simulink model "lugreDenemeFinal"  (R2023b)
settings: Solver=ode23t  StartTime=t_final(1)  StopTime=t_final(end)  FixedStep=1e-3  RelTol=1e-3
values from neighbouring files (symbols this model uses):
  Fc = (v >= 0)*Fc_p + (v < 0)*Fc_n    [frictionModel_20260408.m]    (also in lugreEstTranModel.m = Fc_n; proposed_friction_model.m = params.Fc)
  Fs = (v >= 0)*Fs_p + (v < 0)*Fs_n    [frictionModel_20260408.m]    (also in lugreEstTranModel.m = Fs_n; proposed_friction_model.m = params.Fs)
  vs = vs_n    [lugreEstTranModel.m]    (also in proposed_friction_model.m = params.vs)
undefined symbols (not defined in the file or in its folder): m, sigma_0, sigma_1, sigma_2, v_final
settings Model: Creator=snr  LastModifiedBy=snr

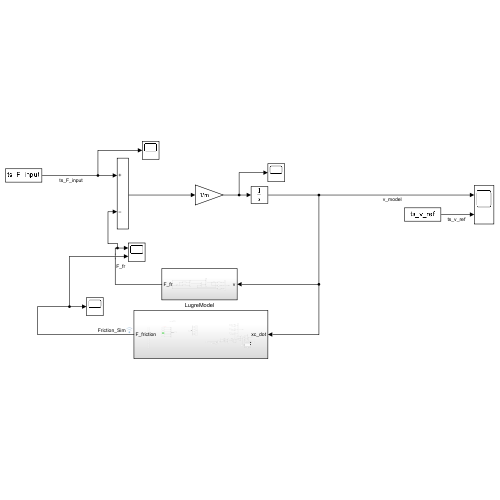
[thumbnail: Simulink's stored preview of the top-level diagram]
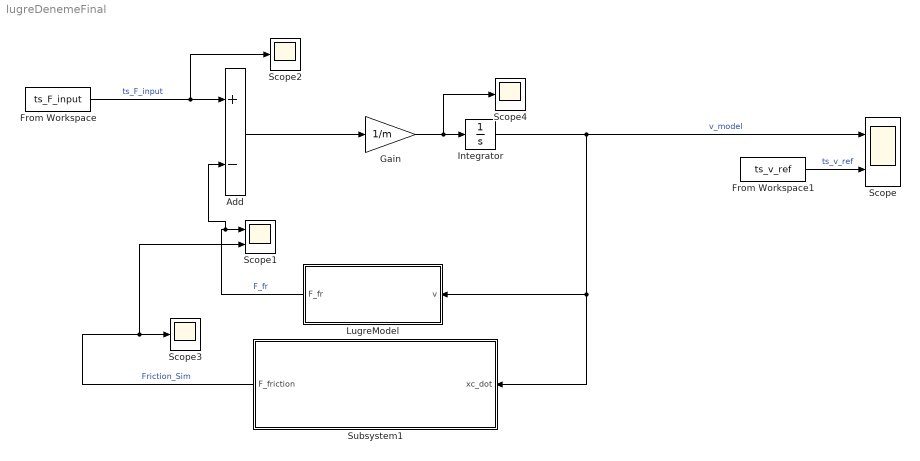
== system lugreDenemeFinal ==
  Add : Sum  Inputs=+-
  From Workspace : FromWorkspace  VariableName=ts_F_input
  From Workspace1 : FromWorkspace  VariableName=ts_v_ref
  Gain : Gain  Gain=1/m
  Integrator : Integrator  InitialCondition=v_final(1)
  LugreModel : Subsystem
  Scope : Scope  NumInputPorts=2
  Scope1 : Scope  NumInputPorts=2
  Scope2 : Scope
  Scope3 : Scope
  Scope4 : Scope
  Subsystem1 : Subsystem
  wires:
  From Workspace/1 -> Scope2/1, Add/1  "ts_F_input"
  Add/1 -> Gain/1
  Gain/1 -> Scope4/1, Integrator/1
  LugreModel/1(F_fr) -> Add/2, Scope1/1  "F_fr"
  Integrator/1 -> Subsystem1/1(xc_dot), LugreModel/1(v), Scope/1  "v_model"
  From Workspace1/1 -> Scope/2  "ts_v_ref"
  Subsystem1/1(F_friction) -> Scope1/2, Scope3/1  "Friction_Sim"

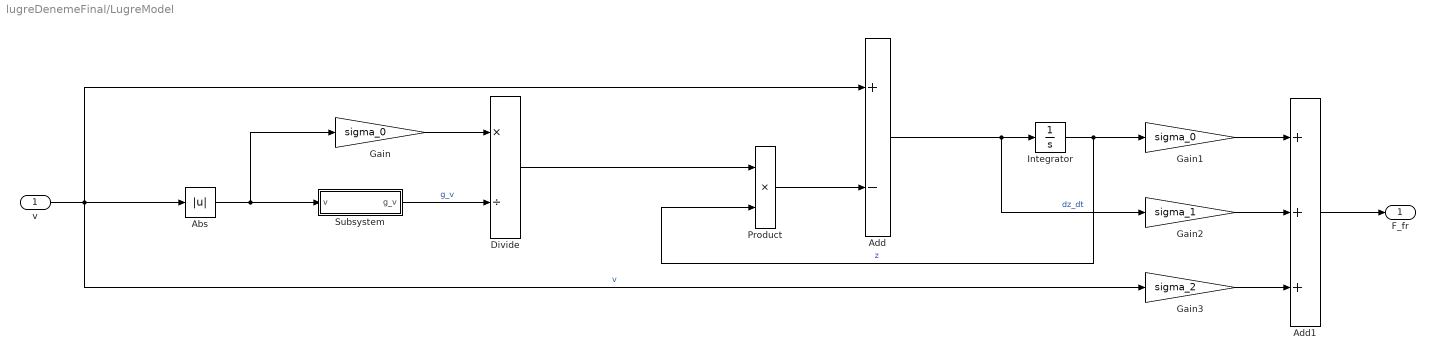
== system lugreDenemeFinal/LugreModel ==
  v : Inport
  Abs : Abs  SaturateOnIntegerOverflow=off
  Add : Sum  Inputs=+-
  Add1 : Sum  Inputs=+++
  Divide : Product  Inputs=*/
  Gain : Gain  Gain=sigma_0
  Gain1 : Gain  Gain=sigma_0
  Gain2 : Gain  Gain=sigma_1
  Gain3 : Gain  Gain=sigma_2
  Integrator : Integrator
  Product : Product
  Subsystem : Subsystem
  F_fr : Outport
  wires:
  v/1 -> Gain3/1, Add/1, Abs/1  "v"
  Abs/1 -> Subsystem/1(v), Gain/1
  Gain/1 -> Divide/1
  Subsystem/1(g_v) -> Divide/2  "g_v"
  Divide/1 -> Product/1
  Integrator/1 -> Gain1/1, Product/2  "z"
  Product/1 -> Add/2
  Add/1 -> Gain2/1, Integrator/1  "dz_dt"
  Gain1/1 -> Add1/1
  Gain2/1 -> Add1/2
  Gain3/1 -> Add1/3
  Add1/1 -> F_fr/1

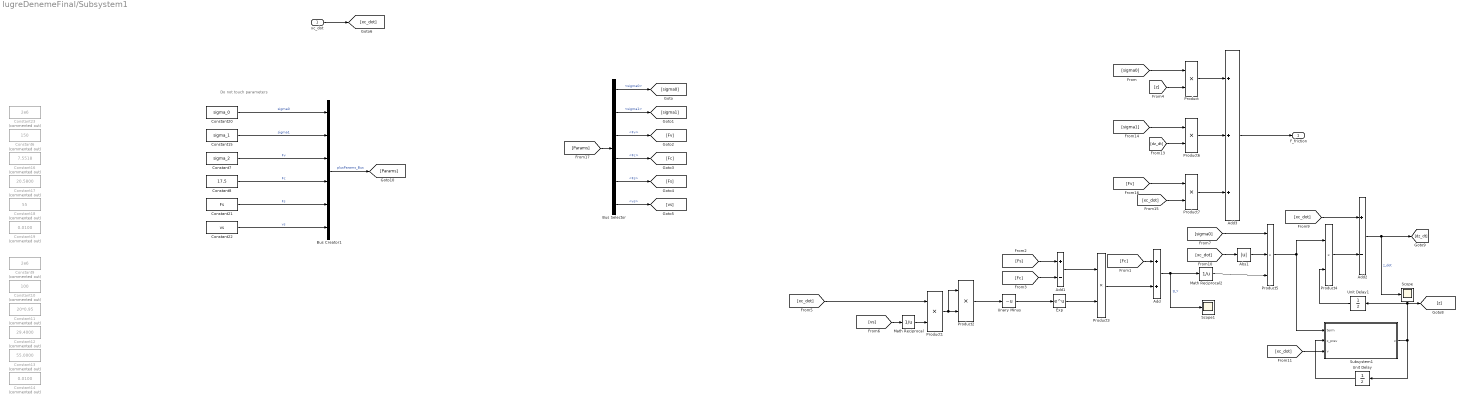
== system lugreDenemeFinal/Subsystem1 ==
  note: Do not touch parameters
  xc_dot : Inport
  Abs1 : Abs  SaturateOnIntegerOverflow=off
  Add : Sum
  Add1 : Sum  Inputs=+-
  Add2 : Sum  Inputs=+-
  Add3 : Sum  Inputs=+++
  Bus Selector : BusSelector  OutputSignals=sigma0,sigma1,Fv,Fc,Fs,vs
  Bus Creator1 : BusCreator  Inputs=6
  Constant10 : Constant  Commented=on  Value=100  OutDataTypeStr=double
  Constant11 : Constant  Commented=on  Value=20*0.95  OutDataTypeStr=double
  Constant12 : Constant  Commented=on  Value=29.4000  OutDataTypeStr=double
  Constant13 : Constant  Commented=on  Value=55.0000  OutDataTypeStr=double
  Constant14 : Constant  Commented=on  Value=0.0100  OutDataTypeStr=double
  Constant15 : Constant  Value=sigma_1  OutDataTypeStr=double
  Constant16 : Constant  Commented=on  Value=7.5518  OutDataTypeStr=double
  Constant17 : Constant  Commented=on  Value=20.5800  OutDataTypeStr=double
  Constant18 : Constant  Commented=on  Value=55  OutDataTypeStr=double
  Constant19 : Constant  Commented=on  Value=0.0100  OutDataTypeStr=double
  Constant20 : Constant  Value=sigma_0  OutDataTypeStr=double
  Constant21 : Constant  Value=Fs  OutDataTypeStr=double
  Constant22 : Constant  Value=vs  OutDataTypeStr=double
  Constant23 : Constant  Commented=on  Value=2e6  OutDataTypeStr=double
  Constant6 : Constant  Commented=on  Value=150  OutDataTypeStr=double
  Constant7 : Constant  Value=sigma_2  OutDataTypeStr=double
  Constant8 : Constant  Value=17.5  OutDataTypeStr=double
  Constant9 : Constant  Commented=on  Value=2e6  OutDataTypeStr=double
  Exp : Math  SignedPower=on
  Math Reciprocal : Math  Operator=reciprocal  SignedPower=on
  Math Reciprocal2 : Math  Operator=reciprocal  SignedPower=on
  Product{,1..4,6..7} (7 alike) : Product
  Product5 : Product  Inputs=3
  Scope : Scope
  Scope1 : Scope
  Subsystem1 : Subsystem
  Unary Minus : UnaryMinus
  Unit Delay : UnitDelay  SampleTime=-1  HasFrameUpgradeWarning=on
  Unit Delay1 : UnitDelay  SampleTime=-1  HasFrameUpgradeWarning=on
  F_friction : Outport
  wires:
  Add3/1 -> F_friction/1
  Product7/1 -> Add3/3
  Product6/1 -> Add3/2
  [Fv] -> Product7/1
  [xc_dot] -> Product7/2
  [dz_dt] -> Product6/2
  [sigma1] -> Product6/1
  Product/1 -> Add3/1
  [z] -> Product/2
  [sigma0] -> Product5/1
  Abs1/1 -> Product5/2
  Add/1 -> Math Reciprocal2/1, Scope1/1  "g_v"
  [xc_dot] -> Abs1/1
  Add1/1 -> Product3/1
  Unary Minus/1 -> Exp/1
  Product2/1 -> Unary Minus/1
  Product1/1 -> Product2/2, Product2/1
  Math Reciprocal/1 -> Product1/2
  [vs] -> Math Reciprocal/1
  [Fc] -> Add1/2
  [Fs] -> Add1/1
  [Fc] -> Add/1
  [sigma0] -> Product/1
  Product3/1 -> Add/2
  Constant20/1 -> Bus Creator1/1  "sigma0"
  Constant15/1 -> Bus Creator1/2  "sigma1"
  Constant22/1 -> Bus Creator1/6  "vs"
  Constant8/1 -> Bus Creator1/4  "Fc"
  Constant7/1 -> Bus Creator1/3  "Fv"
  [Params] -> Bus Selector/1
  Bus Selector/1 -> [sigma0]  "<sigma0>"
  Bus Selector/2 -> [sigma1]  "<sigma1>"
  Bus Selector/3 -> [Fv]  "<Fv>"
  Bus Selector/4 -> [Fc]  "<Fc>"
  Bus Selector/5 -> [Fs]  "<Fs>"
  Bus Selector/6 -> [vs]  "<vs>"
  Math Reciprocal2/1 -> Product5/3
  xc_dot/1 -> [xc_dot]
  Exp/1 -> Product3/2
  Add2/1 -> Scope/1, [dz_dt]  "z_dot"
  [xc_dot] -> Add2/1
  Constant21/1 -> Bus Creator1/5  "Fs"
  Unit Delay1/1 -> Product4/2
  [xc_dot] -> Subsystem1/3(v)
  Subsystem1/1(z) -> [z], Unit Delay1/1, Unit Delay/1
  Unit Delay/1 -> Subsystem1/2(z_prev)
  Product5/1 -> Subsystem1/1(term), Product4/1
  Product4/1 -> Add2/2
  Bus Creator1/1 -> [Params]  "plusParams_Bus"
  [xc_dot] -> Product1/1

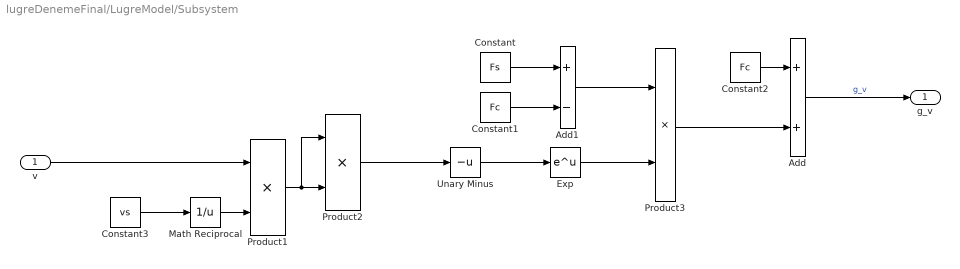
== system lugreDenemeFinal/LugreModel/Subsystem ==
  v : Inport
  Add : Sum
  Add1 : Sum  Inputs=+-
  Constant : Constant  Value=Fs
  Constant1 : Constant  Value=Fc
  Constant2 : Constant  Value=Fc
  Constant3 : Constant  Value=vs
  Exp : Math  SignedPower=on
  Math Reciprocal : Math  Operator=reciprocal  SignedPower=on
  Product1 : Product
  Product2 : Product
  Product3 : Product
  Unary Minus : UnaryMinus
  g_v : Outport
  wires:
  Constant2/1 -> Add/1
  Add/1 -> g_v/1  "g_v"
  Product1/1 -> Product2/2, Product2/1
  Product3/1 -> Add/2
  Constant3/1 -> Math Reciprocal/1
  Exp/1 -> Product3/2
  Math Reciprocal/1 -> Product1/2
  Constant1/1 -> Add1/2
  Add1/1 -> Product3/1
  Product2/1 -> Unary Minus/1
  Unary Minus/1 -> Exp/1
  Constant/1 -> Add1/1
  v/1 -> Product1/1

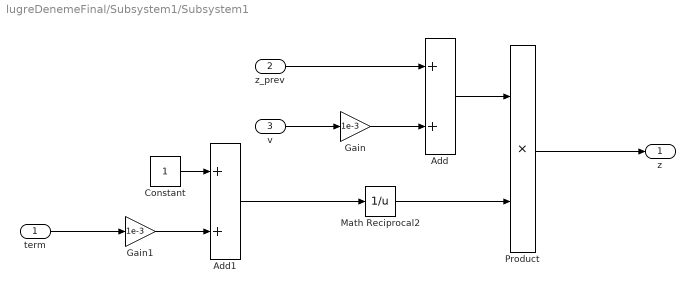
== system lugreDenemeFinal/Subsystem1/Subsystem1 ==
  term : Inport
  z_prev : Inport  Port=2
  v : Inport  Port=3
  Add : Sum
  Add1 : Sum
  Constant : Constant
  Gain : Gain  Gain=1e-3
  Gain1 : Gain  Gain=1e-3
  Math Reciprocal2 : Math  Operator=reciprocal  SignedPower=on
  Product : Product
  z : Outport
  wires:
  term/1 -> Gain1/1
  z_prev/1 -> Add/1
  v/1 -> Gain/1
  Gain/1 -> Add/2
  Add/1 -> Product/1
  Gain1/1 -> Add1/2
  Constant/1 -> Add1/1
  Add1/1 -> Math Reciprocal2/1
  Math Reciprocal2/1 -> Product/2
  Product/1 -> z/1
